simulink subsystem "duty_cycle_allocation_T_P_1"  (R2020b)
settings: Solver=VariableStepAuto  StartTime=0.0  StopTime=10.0  RelTol=1e-3
undefined symbols (not defined in the file): T_P_1, T_P_2
settings Model: Creator=leop9  LastModifiedBy=Previ

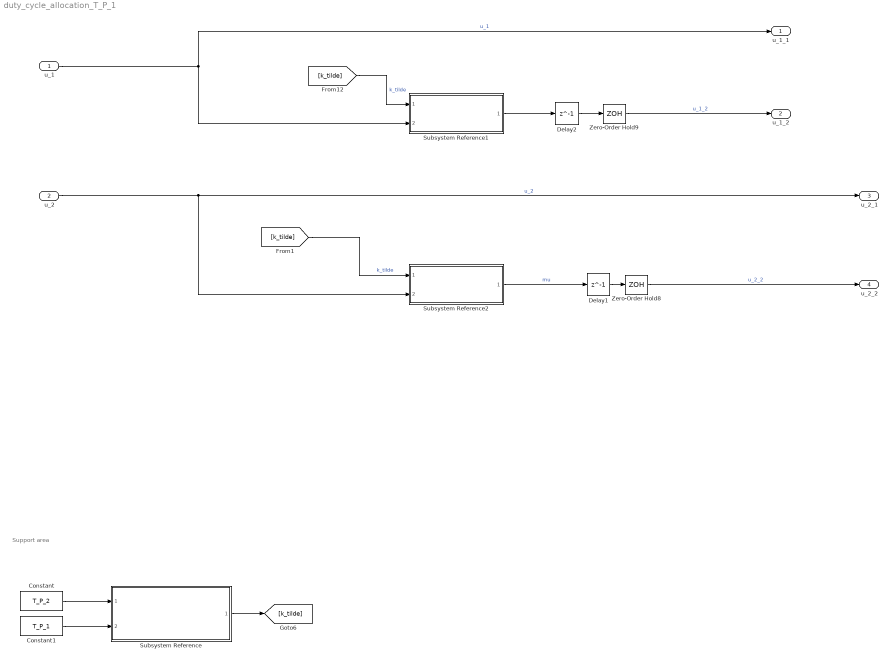
== system duty_cycle_allocation_T_P_1 ==
  note: Support area
  u_1 : Inport
  u_2 : Inport  Port=2
  Constant : Constant  Value=T_P_2
  Constant1 : Constant  Value=T_P_1
  Delay1 : Delay  DelayLength=1  InitialCondition=0
  Delay2 : Delay  DelayLength=1  InitialCondition=0
  Subsystem Reference : Subsystem  ReferencedSubsystem=k_tilde_generator
  Subsystem Reference1 : Subsystem  ReferencedSubsystem=mean_with_reset
  Subsystem Reference2 : Subsystem  ReferencedSubsystem=mean_with_reset
  Zero-Order Hold8 : ZeroOrderHold  SampleTime=T_P_2
  Zero-Order Hold9 : ZeroOrderHold  SampleTime=T_P_2
  u_1_1 : Outport
  u_1_2 : Outport  Port=2
  u_2_1 : Outport  Port=3
  u_2_2 : Outport  Port=4
  wires:
  Subsystem Reference2/1 -> Delay1/1  "mu"
  [k_tilde] -> Subsystem Reference1/1  "k_tilde"
  [k_tilde] -> Subsystem Reference2/1  "k_tilde"
  Subsystem Reference1/1 -> Delay2/1
  u_2/1 -> Subsystem Reference2/2, u_2_1/1  "u_2"
  u_1/1 -> Subsystem Reference1/2, u_1_1/1  "u_1"
  Zero-Order Hold8/1 -> u_2_2/1  "u_2_2"
  Zero-Order Hold9/1 -> u_1_2/1  "u_1_2"
  Delay1/1 -> Zero-Order Hold8/1
  Delay2/1 -> Zero-Order Hold9/1
  Constant/1 -> Subsystem Reference/1
  Subsystem Reference/1 -> [k_tilde]
  Constant1/1 -> Subsystem Reference/2
